simulink model "Playground"  (R2015b)
settings: Solver=VariableStepAuto  StartTime=0.0  StopTime=10.0  FixedStep=10/1024  RelTol=1e-3
undefined symbols (not defined in the file or in its folder): sigbuilder_block
libraries: fl_lib x19, nesl_utility x3
settings Model: Creator=OlgeirMac  LastModifiedBy=OlgeirMac

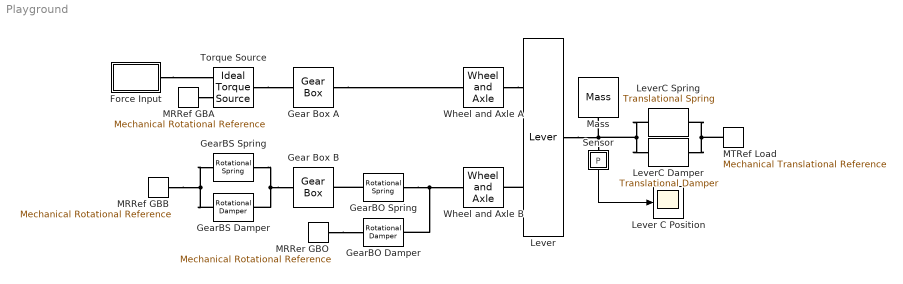
== system Playground ==
  Force Input : Subsystem
  Gear Box A : fl_lib/Mechanical/Mechanisms/Gear Box  Tag=Factory Generic  ratio=4  t_in_specify=off  t_in_priority=High  t_in=0 N*m  t_out_specify=off  t_out_priority=High  t_out=0 N*m
  Gear Box B : fl_lib/Mechanical/Mechanisms/Gear Box  Tag=Factory Generic  ratio=2  t_in_specify=off  t_in_priority=High  t_in=0 N*m  t_out_specify=off  t_out_priority=High  t_out=0 N*m
  GearBO Damper : fl_lib/Mechanical/Rotational Elements/Rotational Damper  Tag=Factory Generic  D=0.0004 m*s*N/rad  w_specify=off  w_priority=High  w=0 rad/s  t_specify=off  t_priority=High  t=0 N*m
  GearBO Spring : fl_lib/Mechanical/Rotational Elements/Rotational Spring  Tag=Factory Generic  spr_rate=100 m*N/rad  w_specify=off  w_priority=High  w=0 rad/s  t_specify=off  t_priority=High  t=0 N*m  phi_specify=on  phi_priority=High  phi=0 rad
  GearBS Damper : fl_lib/Mechanical/Rotational Elements/Rotational Damper  Tag=Factory Generic  D=0.0006 m*s*N/rad  w_specify=off  w_priority=High  w=0 rad/s  t_specify=off  t_priority=High  t=0 N*m
  GearBS Spring : fl_lib/Mechanical/Rotational Elements/Rotational Spring  Tag=Factory Generic  spr_rate=100 m*N/rad  w_specify=off  w_priority=High  w=0 rad/s  t_specify=off  t_priority=High  t=0 N*m  phi_specify=on  phi_priority=High  phi=0 rad
  Lever : fl_lib/Mechanical/Mechanisms/Lever  Tag=Factory Generic  arm_AC=0.1 m  arm_BC=0.1 m  f_A_specify=off  f_A_priority=High  f_A=0 N  f_B_specify=off  f_B_priority=High  f_B=0 N  f_C_specify=off  f_C_priority=High  f_C=0 N
  Lever C Position : Scope
  LeverC Damper : fl_lib/Mechanical/Translational Elements/Translational Damper  Tag=Factory Generic  D=64 s*N/m  v_specify=off  v_priority=High  v=0 m/s  f_specify=off  f_priority=High  f=0 N
  LeverC Spring : fl_lib/Mechanical/Translational Elements/Translational Spring  Tag=Factory Generic  spr_rate=10000 N/m  v_specify=off  v_priority=High  v=0 m/s  f_specify=off  f_priority=High  f=0 N  x_specify=on  x_priority=High  x=0 m
  MRRef GBA : fl_lib/Mechanical/Rotational Elements/Mechanical Rotational Reference  Tag=Factory Generic
  MRRef GBB : fl_lib/Mechanical/Rotational Elements/Mechanical Rotational Reference  Tag=Factory Generic
  MRRer GBO : fl_lib/Mechanical/Rotational Elements/Mechanical Rotational Reference  Tag=Factory Generic
  MTRef Load : fl_lib/Mechanical/Translational Elements/Mechanical Translational Reference  Tag=Factory Generic
  Mass : fl_lib/Mechanical/Translational Elements/Mass  Tag=Factory Generic  mass=120 kg  v_specify=on  v_priority=High  v=0 m/s  f_specify=off  f_priority=High  f=0 N
  Sensor : Subsystem
      mask Display: disp('P')
  Torque Source : fl_lib/Mechanical/Mechanical Sources/Ideal Torque Source  Tag=Factory Generic
  Wheel and Axle A : fl_lib/Mechanical/Mechanisms/Wheel and Axle  Tag=Factory Generic  R=0.05 m  or=1  orient=1  t_specify=off  t_priority=High  t=0 N*m  f_specify=off  f_priority=High  f=0 N
  Wheel and Axle B : fl_lib/Mechanical/Mechanisms/Wheel and Axle  Tag=Factory Generic  R=0.8 m  or=1  orient=1  t_specify=off  t_priority=High  t=0 N*m  f_specify=off  f_priority=High  f=0 N
  wires:
  Sensor/1(P) -> Lever C Position/1
  connections:
  LeverC Damper/LConn1 -- LeverC Spring/LConn1 -- Lever/RConn1 -- Sensor/LConn1 -- Mass/LConn1
  LeverC Spring/RConn1 -- MTRef Load/LConn1 -- LeverC Damper/RConn1
  GearBS Spring/LConn1 -- MRRef GBB/LConn1 -- GearBS Damper/RConn1
  Gear Box B/LConn1 -- GearBS Spring/RConn1 -- GearBS Damper/LConn1
  GearBO Damper/LConn1 -- GearBO Spring/RConn1 -- Wheel and Axle B/LConn1
  Torque Source/LConn1 -- Gear Box A/LConn1
  MRRef GBA/LConn1 -- Torque Source/RConn2
  GearBO Spring/LConn1 -- Gear Box B/RConn1
  MRRer GBO/LConn1 -- GearBO Damper/RConn1
  Force Input/RConn1 -- Torque Source/RConn1
  Gear Box A/RConn1 -- Wheel and Axle A/LConn1
  Wheel and Axle A/RConn1 -- Lever/LConn1
  Lever/LConn2 -- Wheel and Axle B/RConn1

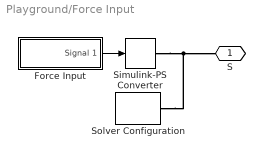
== system Playground/Force Input ==
  Force Input : Subsystem  Tag=STV Subsys  LoadFcn=sigbuilder_block('load');  StartFcn=sigbuilder_block('start');  StopFcn=sigbuilder_block('stop');  ClipboardFcn=sigbuilder_block('clipboard');  mask(Sigbuilder block){}
      mask help: Sigbuilder GUI
      mask init:
      | if ~strcmp(get_param(bdroot(gcbh),'SimulationStatus'),'stopped') tuvar = sigbuilder_block('maskInit'); end
      settings: CopyFcn=sigbuilder_block('copy');  DeleteFcn=sigbuilder_block('delete');  ModelCloseFcn=sigbuilder_block('modelClose');  PreSaveFcn=sigbuilder_block('preSave');  PauseFcn=sigbuilder_block('pause')  ContinueFcn=sigbuilder_block('continue')  NameChangeFcn=sigbuilder_block('namechange');  OpenFcn=sigbuilder_block('open',[622 195 527 253 ]);  CloseFcn=sigbuilder_block('close');
      mask Display: plot(0,0,100,100,[10,10,40,40,10],[80,20,20,80,80],[40,10],[50,50], [40,27,10],[65,72,56],[40,25,25,10],[28,28,43,43]);
  Simulink-PS Converter : nesl_utility/Simulink-PS Converter  PhysicalDomain=network_engine_domain  SubClassName=ps_input  LeftPortType=input  RightPortType=output  PseudoPeriodic=off  Frequencies=[]  NoiseDistribution=none  NoiseParameters=[]  Unit=1  AffineConversion=off  InputFiltering=off  SimscapeFilterOrder=1  InputFilterTimeConstant=.001  UdotUserProvided=[]
  Solver Configuration : nesl_utility/Solver Configuration  PhysicalDomain=network_engine_domain  SubClassName=solver  LeftPortType=input  RightPortType=generic  Accelerate=off  Tones=[]  Harmonics=[]  SimulateNoise=off  Profile=off  UseLocalSampling=off  EnableSwitchedLinearOptims=on  FrequencyDomain=off  UseCCode=off  RelTol=0.001  AbsTol=1e-06  MinStep=1e-09  ToWorkspace=off  RevertToSquareIcSolve=off  NumHomotopyIterations=100  PhasorMode=off  PhasorModeNumHarmonics=1  DoDC=off  ResidualTolerance=1e-9  UseLocalSolver=off  LocalSolverChoice=NE_BACKWARD_EULER_ADVANCER  LocalSolverSampleTime=.001  DoFixedCost=off  MaxNonlinIter=3  MaxModeIter=2  LinearAlgebra=Sparse  DelaysMemoryBudget=1024  AutomaticFiltering=on  FilteringTimeConstant=0.001
  S : PMIOPort  Port=1  Side=Right
  wires:
  Force Input/1(Signal 1) -> Simulink-PS Converter/1
  connections:
  Simulink-PS Converter/RConn1 -- Solver Configuration/RConn1 -- S/RConn1

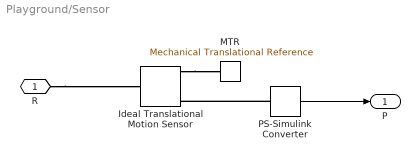
== system Playground/Sensor ==
  Ideal Translational Motion Sensor : fl_lib/Mechanical/Mechanical Sensors/Ideal Translational Motion Sensor  Tag=Factory Generic  offset=0 m
  MTR : fl_lib/Mechanical/Translational Elements/Mechanical Translational Reference  Tag=Factory Generic
  PS-Simulink Converter : nesl_utility/PS-Simulink Converter  PhysicalDomain=network_engine_domain  SubClassName=ps_output  LeftPortType=input  RightPortType=output  PseudoPeriodic=off  Frequencies=[]  Unit=1  AffineConversion=off
  R : PMIOPort  Port=1  Side=Left
  P : Outport
  wires:
  PS-Simulink Converter/1 -> P/1
  connections:
  Ideal Translational Motion Sensor/RConn1 -- MTR/LConn1
  PS-Simulink Converter/LConn1 -- Ideal Translational Motion Sensor/RConn3
  R/RConn1 -- Ideal Translational Motion Sensor/LConn1

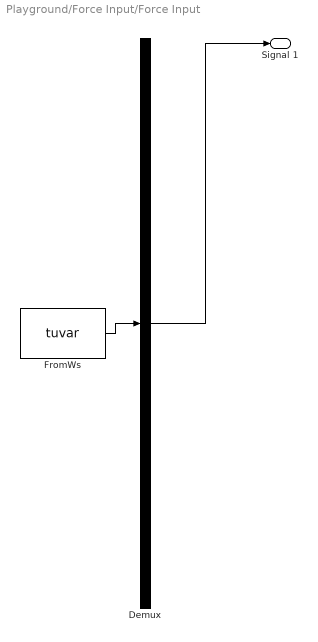
== system Playground/Force Input/Force Input ==
  Demux : Demux  Tag=STV Demux  Outputs=1
  FromWs : FromWorkspace  Tag=STV FromWs  VariableName=tuvar  SampleTime=0
      SigBuilderData=|
      | common.afterFinalStr = 'Extrapolate'
      | common.sampleTime = 0
      | dataSet.timeRange = [0 10]
      | dataSet.name = 'Group 1'
      | sbobj.Groups.Name = 'Group 1'
      | sbobj.Groups.Signals.Name = 'Signal 1'
      | sbobj.Groups.Signals.XData = [0 0.2 0.34 0.34 3 3 3.22 6 6.2 10]
      | sbobj.Groups.Signals.YData = [0 0 12 7 5 2 -12 -12 0 0]
  Signal 1 : Outport  Tag=STV Outport
  wires:
  Demux/1 -> Signal 1/1
  FromWs/1 -> Demux/1
